simulink model "TestDyn_4CIGs_OP_7_LIN"  (R2024b)
settings: Solver=ode45  StartTime=0.0  StopTime=Tsim_lin  RelTol=1e-3
undefined symbols (not defined in the file): delta_u, sim_config, ss_sys, tstep_lin
settings Model: Creator=Francesca  LastModifiedBy=Francesca

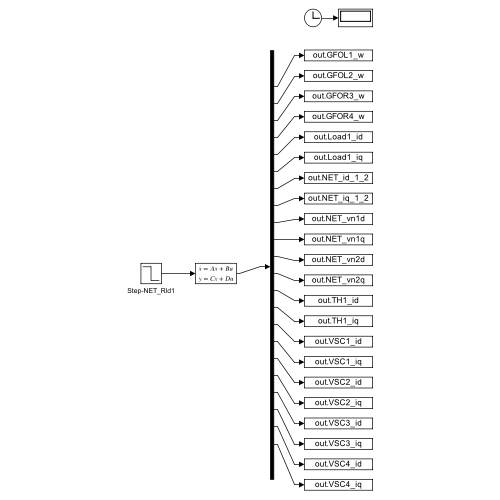
[thumbnail: Simulink's stored preview of the top-level diagram]
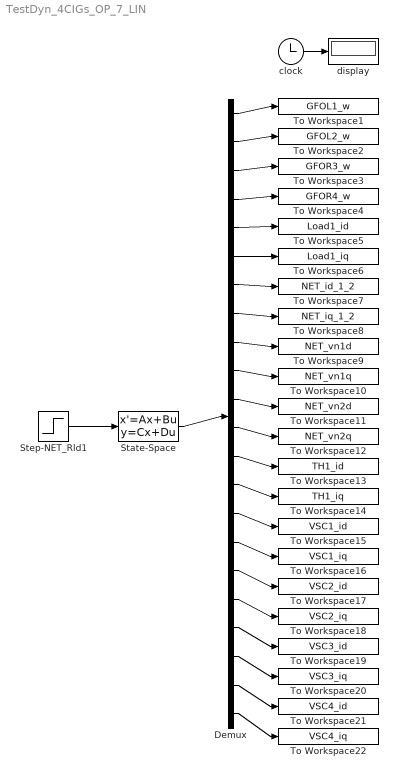
== system TestDyn_4CIGs_OP_7_LIN ==
  Demux : Demux  Outputs=22
  State-Space : StateSpace  A=ss_sys.A  B=ss_sys.B  C=ss_sys.C  D=ss_sys.D  InitialCondition=0
  Step-NET_Rld1 : Step  Time=tstep_lin  After=delta_u  SampleTime=0
  To Workspace1 : ToWorkspace  VariableName=GFOL1_w  SampleTime=sim_config.Tsample
  To Workspace10 : ToWorkspace  VariableName=NET_vn1q  SampleTime=sim_config.Tsample
  To Workspace11 : ToWorkspace  VariableName=NET_vn2d  SampleTime=sim_config.Tsample
  To Workspace12 : ToWorkspace  VariableName=NET_vn2q  SampleTime=sim_config.Tsample
  To Workspace13 : ToWorkspace  VariableName=TH1_id  SampleTime=sim_config.Tsample
  To Workspace14 : ToWorkspace  VariableName=TH1_iq  SampleTime=sim_config.Tsample
  To Workspace15 : ToWorkspace  VariableName=VSC1_id  SampleTime=sim_config.Tsample
  To Workspace16 : ToWorkspace  VariableName=VSC1_iq  SampleTime=sim_config.Tsample
  To Workspace17 : ToWorkspace  VariableName=VSC2_id  SampleTime=sim_config.Tsample
  To Workspace18 : ToWorkspace  VariableName=VSC2_iq  SampleTime=sim_config.Tsample
  To Workspace19 : ToWorkspace  VariableName=VSC3_id  SampleTime=sim_config.Tsample
  To Workspace2 : ToWorkspace  VariableName=GFOL2_w  SampleTime=sim_config.Tsample
  To Workspace20 : ToWorkspace  VariableName=VSC3_iq  SampleTime=sim_config.Tsample
  To Workspace21 : ToWorkspace  VariableName=VSC4_id  SampleTime=sim_config.Tsample
  To Workspace22 : ToWorkspace  VariableName=VSC4_iq  SampleTime=sim_config.Tsample
  To Workspace3 : ToWorkspace  VariableName=GFOR3_w  SampleTime=sim_config.Tsample
  To Workspace4 : ToWorkspace  VariableName=GFOR4_w  SampleTime=sim_config.Tsample
  To Workspace5 : ToWorkspace  VariableName=Load1_id  SampleTime=sim_config.Tsample
  To Workspace6 : ToWorkspace  VariableName=Load1_iq  SampleTime=sim_config.Tsample
  To Workspace7 : ToWorkspace  VariableName=NET_id_1_2  SampleTime=sim_config.Tsample
  To Workspace8 : ToWorkspace  VariableName=NET_iq_1_2  SampleTime=sim_config.Tsample
  To Workspace9 : ToWorkspace  VariableName=NET_vn1d  SampleTime=sim_config.Tsample
  clock : Clock
  display : Display
  wires:
  clock/1 -> display/1
  Step-NET_Rld1/1 -> State-Space/1
  State-Space/1 -> Demux/1
  Demux/1 -> To Workspace1/1
  Demux/2 -> To Workspace2/1
  Demux/3 -> To Workspace3/1
  Demux/4 -> To Workspace4/1
  Demux/5 -> To Workspace5/1
  Demux/6 -> To Workspace6/1
  Demux/7 -> To Workspace7/1
  Demux/8 -> To Workspace8/1
  Demux/9 -> To Workspace9/1
  Demux/10 -> To Workspace10/1
  Demux/11 -> To Workspace11/1
  Demux/12 -> To Workspace12/1
  Demux/13 -> To Workspace13/1
  Demux/14 -> To Workspace14/1
  Demux/15 -> To Workspace15/1
  Demux/16 -> To Workspace16/1
  Demux/17 -> To Workspace17/1
  Demux/18 -> To Workspace18/1
  Demux/19 -> To Workspace19/1
  Demux/20 -> To Workspace20/1
  Demux/21 -> To Workspace21/1
  Demux/22 -> To Workspace22/1
